simulink model "PLL"  (R2022b)
settings: Solver=VariableStepAuto  StartTime=0.0  StopTime=1000  RelTol=1e-3
libraries: commrandsrc3 x1, simulink x1, commdigbbndpm3 x1
settings Model: Creator=f3d3r  LastModifiedBy=f3d3r
settings DebuggingCC: UnconnectedInputMsg=warning  UnconnectedOutputMsg=warning  UnconnectedLineMsg=warning
settings ModelReferenceCC: EnableRefExpFcnMdlSchedulingChecks=on
settings RTWCC: DLArmComputeVersion=19.05

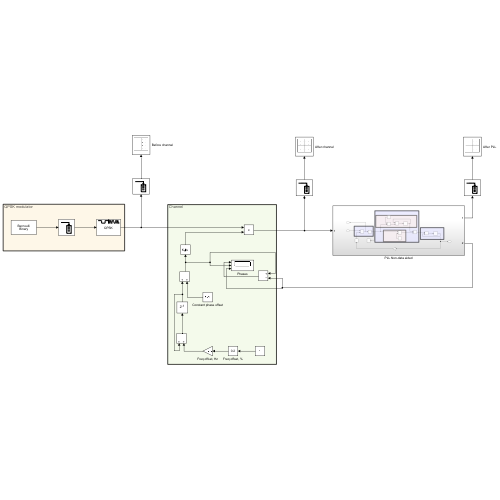
[thumbnail: Simulink's stored preview of the top-level diagram]
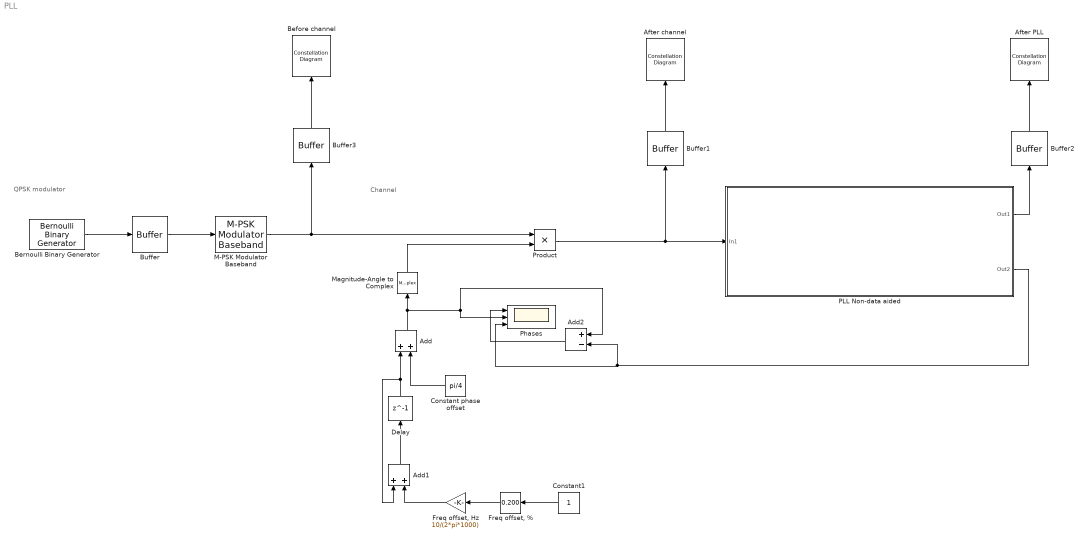
== system PLL ==
  note: Channel
  note: QPSK modulator
  Add : Sum
  Add1 : Sum
  Add2 : Sum  Inputs=+-
  After PLL : ConstellationDiagram  WindowPosition=[999.000000,596.000000,476.000000,454.000000,]  Visible=on  ScopeFrameLocation=window  ShowReferenceConstellation=off  DefaultConfigurationName=comm.scopes.ConstellationDiagramBlockCfg
  After channel : ConstellationDiagram  WindowPosition=[1472.000000,2.000000,448.000000,562.000000,]  Visible=on  ScopeFrameLocation=window  ShowReferenceConstellation=off  DefaultConfigurationName=comm.scopes.ConstellationDiagramBlockCfg
  Before channel : ConstellationDiagram  WindowPosition=[1473.000000,596.000000,452.000000,454.000000,]  Visible=on  ScopeFrameLocation=window  XLimits=[-0.94638 0.94638]  YLimits=[-0.94638 0.94638]  ShowReferenceConstellation=off  DefaultConfigurationName=comm.scopes.ConstellationDiagramBlockCfg
  Bernoulli Binary Generator : commrandsrc3/Bernoulli Binary Generator  ProbabilityOfZero=0.5  SeedSource=Auto  Seed=0  SampleTime=1/1000  SamplesPerFrame=1  OutputDataType=double  SimulateUsing=Interpreted execution
  Buffer : Buffer  N=2  OutputFrames=off
  Buffer1 : Buffer  N=9000  OutputFrames=off
  Buffer2 : Buffer  N=1024  OutputFrames=off
  Buffer3 : Buffer  N=1024  OutputFrames=off
  Constant phase offset : Constant  Value=pi/4
  Constant1 : Constant
  Delay : Delay  DelayLength=1
  "Freq offset, %" : simulink/Math Operations/Slider Gain  gain=0.200  low=0  high=0.2
  "Freq offset, Hz" : Gain  Gain=10/(2*pi*1000)
  M-PSK Modulator Baseband : commdigbbndpm3/M-PSK Modulator Baseband  M=4  InType=Bit  Enc=Gray  Mapping=[0:7]  Ph=pi/4  outDtype=double  outWordLen=16  outUDDataType=sfix(16)  outFracLenMode=Best precision  outFracLen=15  outDataTypeStr=double  outLastDataTypeStr=double
  Magnitude-Angle to Complex : MagnitudeAngleToComplex  Input=Angle  ConstantPart=1
  PLL Non-data aided : Subsystem
  Phases : Scope  NumInputPorts=3
  Product : Product
  wires:
  Bernoulli Binary Generator/1 -> Buffer/1
  Buffer/1 -> M-PSK Modulator Baseband/1
  Buffer1/1 -> After channel/1
  Product/1 -> Buffer1/1, PLL Non-data aided/1(In1)
  Magnitude-Angle to Complex/1 -> Product/2
  Add/1 -> Phases/2, Add2/1, Magnitude-Angle to Complex/1
  Constant phase offset/1 -> Add/2
  Add1/1 -> Delay/1
  Delay/1 -> Add/1, Add1/1
  "Freq offset, %"/1 -> "Freq offset, Hz"/1
  "Freq offset, Hz"/1 -> Add1/2
  Constant1/1 -> "Freq offset, %"/1
  Buffer2/1 -> After PLL/1
  PLL Non-data aided/1(Out1) -> Buffer2/1
  M-PSK Modulator Baseband/1 -> Buffer3/1, Product/1
  Buffer3/1 -> Before channel/1
  PLL Non-data aided/2(Out2) -> Phases/3, Add2/2
  Add2/1 -> Phases/1

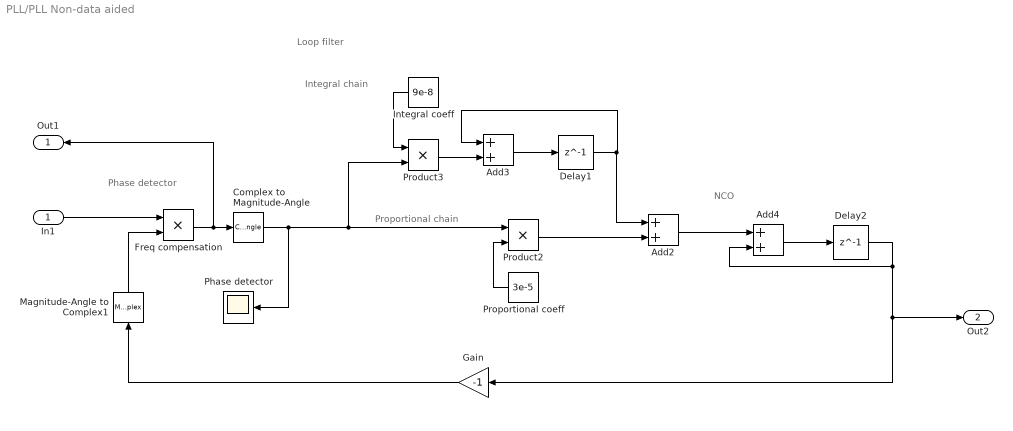
== system PLL/PLL Non-data aided ==
  note: Integral chain
  note: Phase detector
  note: Loop filter
  note: NCO
  note: Proportional chain
  In1 : Inport
  Add2 : Sum
  Add3 : Sum
  Add4 : Sum
  Complex to Magnitude-Angle : ComplexToMagnitudeAngle  Output=Angle
  Delay1 : Delay  DelayLength=1
  Delay2 : Delay  DelayLength=1
  Freq compensation : Product
  Gain : Gain  Gain=-1
  Integral coeff : Constant  Value=9e-8
  Magnitude-Angle to Complex1 : MagnitudeAngleToComplex  Input=Angle  ConstantPart=1
  Phase detector : Scope
  Product2 : Product
  Product3 : Product
  Proportional coeff : Constant  Value=3e-5
  Out1 : Outport
  Out2 : Outport  Port=2
  wires:
  Integral coeff/1 -> Product3/1
  Delay1/1 -> Add2/1, Add3/1
  Complex to Magnitude-Angle/1 -> Product3/2, Product2/1, Phase detector/1
  Add4/1 -> Delay2/1
  Freq compensation/1 -> Out1/1, Complex to Magnitude-Angle/1
  Add3/1 -> Delay1/1
  Delay2/1 -> Add4/2, Gain/1, Out2/1
  In1/1 -> Freq compensation/1
  Magnitude-Angle to Complex1/1 -> Freq compensation/2
  Product2/1 -> Add2/2
  Add2/1 -> Add4/1
  Proportional coeff/1 -> Product2/2
  Product3/1 -> Add3/2
  Gain/1 -> Magnitude-Angle to Complex1/1
